simulink model "RoboBoat_SScall"  (R2014a)
settings: Solver=FixedStepDiscrete  StartTime=0.0  StopTime=inf  FixedStep=.25  RelTol=1e-3
undefined symbols (not defined in the file): Com1, Com2, Com3, Com4, DiscIntNeverNeededParam, standard
libraries: xpcseriallib x31, visiontextngfix x25, simulink x19, slrtlib x9, speedgoatlib_IO102 x3, speedgoatlib x1
(part 5 of 5)

== matlab function RoboBoat_SScall/Sensors/1020 Comms/MATLAB Function3 ==
  data: Time input; asciiHRT output; Lat input; Long input; Mode input; Task input
% This function creates the heartbeat message to be sent from Speedgoat in
% ascii code
% Written by: Edward Zhu
% Date: 9/17/14

function asciiHRT = asciiHRTEncoder(Time, Lat, Long, Mode, Task)

% Initialize output message vector as the serial output block expects 128
% character message
asciiHRT = uint8(zeros(1,128));

% Convert static strings to ascii code
asciiMsgID = uint8('$RXHRT,');
asciiComma = uint8(',');
asciiDeciPt = uint8('.');
if Lat >= 0
    asciiNS = uint8('N,');
else
    Lat = -Lat;
    asciiNS = uint8('S,');
end
if Long >= 0
    asciiEW = uint8('E,');
else
    Long = -Long;
    asciiEW = uint8('W,');
end
asciiTeamID = uint8('FAUVU,');
asciiMsgEnd = uint8('*');
asciiMsgCRLF = [13 10];

% Convert UTC Time input (hhmmss) into ascii code
asciiTime = uint8(zeros(1,7));
asciiTime(7) = asciiComma;

for timeChar = 1:6
    asciiTime(timeChar) = floor(mod(Time,10^(7-timeChar))/...
        10^(6-timeChar)) + 48;
end

% Convert latitude (dd.mmmmmm) into ascii code
asciiLat = uint8(zeros(1,10));
asciiLat(10) = asciiComma;
asciiLat(3) = asciiDeciPt;

latInt = floor(Lat);
for latIntChar = 1:2
    asciiLat(latIntChar) = floor(mod(latInt,10^(3-latIntChar))/...
        10^(2-latIntChar)) + 48;
end

latDeci = mod(Lat,latInt) * 10^6;
for latDeciChar = 1:6
    asciiLat(latDeciChar+3) = floor(mod(latDeci,10^(7-latDeciChar))/...
        10^(6-latDeciChar)) + 48;
end

% Convert longitude (ddd.mmmmmm) into ascii code
asciiLong = uint8(zeros(1,11));
asciiLong(11) = asciiComma;
asciiLong(4) = asciiDeciPt;

longInt = floor(Long);
for longIntChar = 1:3
    asciiLong(longIntChar) = floor(mod(longInt,10^(4-longIntChar))/...
        10^(3-longIntChar)) + 48;
end

longDeci = mod(Long,longInt) * 10^6;
for longDeciChar = 1:6
    asciiLong(longDeciChar+4) = floor(mod(longDeci,10^(7-longDeciChar))/...
        10^(6-longDeciChar)) + 48;
end

% Convert vehicle mode into ascii (1 = RC, 2 = Auto)
if Mode ~= 1 || Mode ~= 2
    Mode = 1;
    asciiMode = [uint8(Mode+48) asciiComma];
else
    asciiMode = [uint8(Mode+48) asciiComma];
end

% Convert vehicle task into ascii
asciiTask = [uint8(Task+48) asciiMsgEnd];

% Concat individual ascii arrays into one array
asciiPreChkSum = cat(2,asciiMsgID,asciiTime,asciiLat,asciiNS,asciiLong,asciiEW,...
    asciiTeamID,asciiMode,asciiTask);

% Calculate the checksum of the message from the '$' to the '*' and convert
% to hex
chkSum = uint8(0);

for chksumChar = 1:(length(asciiPreChkSum)-2)
    chkSum = bitxor(chkSum,asciiPreChkSum(chksumChar+1));
end

% Convert the checksum to ascii
chkSum = dec2hex(chkSum);
asciiChkSum = uint8(zeros(1,length(chkSum))+32);
for i = 1:length(chkSum)
    asciiChkSum(i) = uint8(chkSum(i));
end

% Concat the checksum and the '/r/n' to the end of the message
asciiPostChkSum = cat(2,asciiPreChkSum,asciiChkSum,asciiMsgCRLF);

% Output the final message
asciiHRT(1:length(asciiPostChkSum)) = asciiPostChkSum;
